simulink model "observer_CT_simulink"  (R2022b)
settings: Solver=VariableStepAuto  StartTime=0.0  StopTime=10.0  RelTol=1e-3
undefined symbols (not defined in the file): A, Ahat, amplitude, B, Bhat, C, Chat, D, Dhat, freq, initpha, x0, xhat0
settings Model: Creator=tpjch  LastModifiedBy=xuchen

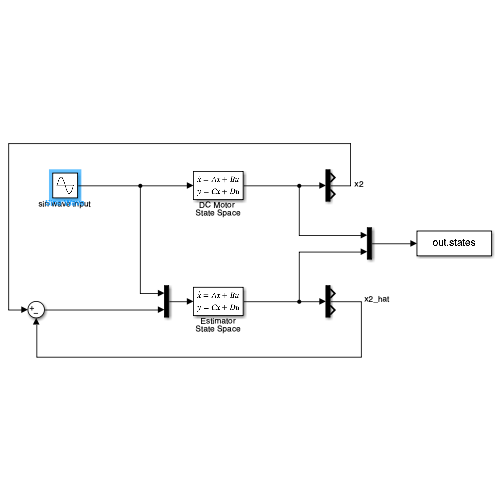
[thumbnail: Simulink's stored preview of the top-level diagram]
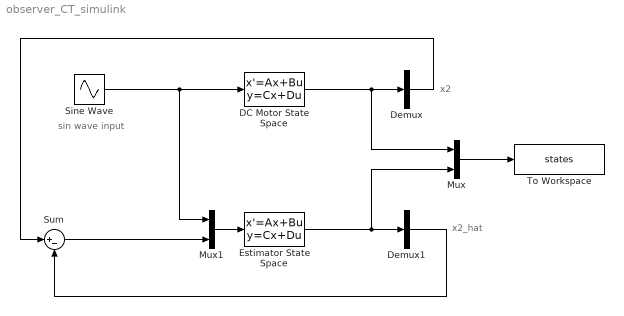
== system observer_CT_simulink ==
  note: x2
  note: x2_hat
  note: sin wave input
  DC Motor State Space : StateSpace  A=A  B=B  C=C  D=D  InitialCondition=x0
  Demux : Demux  Outputs=3
  Demux1 : Demux  Outputs=3
  Estimator State Space : StateSpace  A=Ahat  B=Bhat  C=Chat  D=Dhat  InitialCondition=xhat0
  Mux : Mux  Inputs=2
  Mux1 : Mux  Inputs=2
  Sine Wave : Sin  Amplitude=amplitude  Frequency=freq  Phase=initpha  SampleTime=0
  Sum : Sum  Inputs=|+-
  To Workspace : ToWorkspace  VariableName=states  SaveFormat=Timeseries  SampleTime=-1
  wires:
  DC Motor State Space/1 -> Demux/1, Mux/1
  Mux/1 -> To Workspace/1
  Estimator State Space/1 -> Demux1/1, Mux/2
  Sine Wave/1 -> Mux1/1, DC Motor State Space/1
  Mux1/1 -> Estimator State Space/1
  Sum/1 -> Mux1/2
  Demux1/2 -> Sum/2
  Demux/2 -> Sum/1
